simulink subsystem "VL53L_Sensor"  (R2022b)
settings: Solver=VariableStepAuto  StartTime=0.0  StopTime=10.0  RelTol=1e-3
undefined symbols (not defined in the file): K_cc, x
libraries: arduinosensorlib x2
settings Model: Creator=dar.io  LastModifiedBy=dar.io

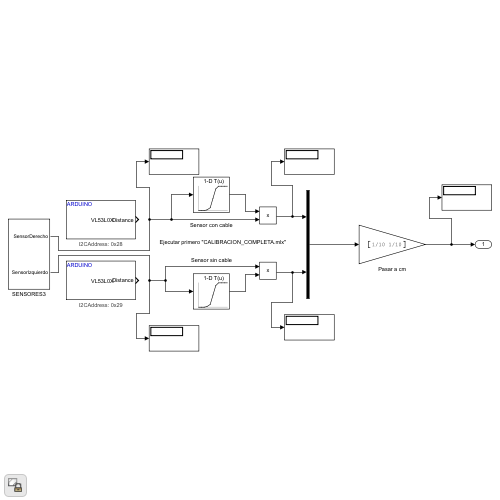
[thumbnail: Simulink's stored preview of the top-level diagram]
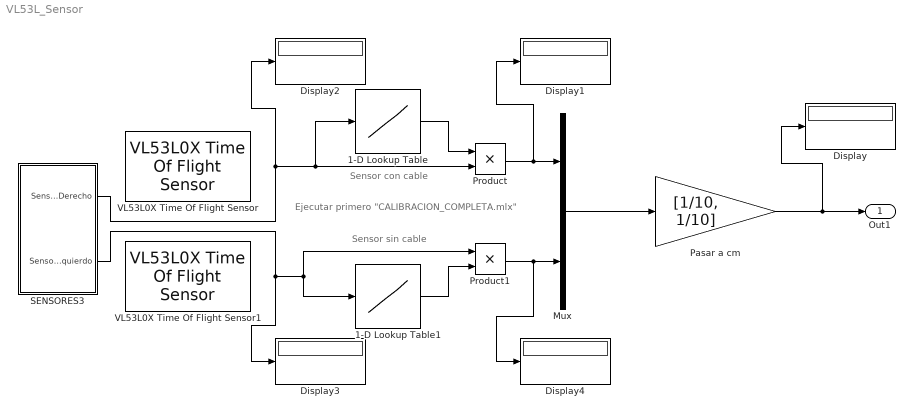
== system VL53L_Sensor ==
  note: Ejecutar primero "CALIBRACION_COMPLETA.mlx"
  note: Sensor sin cable
  note: Sensor con cable
  1-D Lookup Table : Lookup_n-D  NumberOfTableDimensions=1  BreakpointsForDimension1=x  Table=K_cc  ExtrapMethod=Clip  InternalRulePriority=Speed  RndMeth=Simplest
  1-D Lookup Table1 : Lookup_n-D  NumberOfTableDimensions=1  BreakpointsForDimension1=x  Table=K_cc  ExtrapMethod=Clip  InternalRulePriority=Speed  RndMeth=Simplest
  Display{,1..4} (5 alike) : Display
  Mux : Mux  Inputs=2
  Pasar a cm : Gain  Gain=[1/10, 1/10]
  Product : Product
  Product1 : Product
  SENSORES3 : Subsystem
  VL53L0X Time Of Flight Sensor : arduinosensorlib/VL53L0X Time Of Flight Sensor  I2CAddress=0x28  BitRate=1000000  RangingMode=Default  SampleTime=-1
      settings: AttributesFormatString=I2CAddress: %<I2CAddress>
  VL53L0X Time Of Flight Sensor1 : arduinosensorlib/VL53L0X Time Of Flight Sensor  I2CAddress=0x29  BitRate=1000000  RangingMode=Default  SampleTime=-1
      settings: AttributesFormatString=I2CAddress: %<I2CAddress>
  Out1 : Outport
  wires:
  Mux/1 -> Pasar a cm/1
  Pasar a cm/1 -> Out1/1, Display/1
  1-D Lookup Table/1 -> Product/1
  1-D Lookup Table1/1 -> Product1/2
  Product/1 -> Display1/1, Mux/1
  SENSORES3/1(SensorDerecho) -> Display2/1, Product/2, 1-D Lookup Table/1
  SENSORES3/2(SensorIzquierdo) -> 1-D Lookup Table1/1, Product1/1, Display3/1
  Product1/1 -> Display4/1, Mux/2

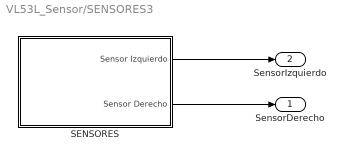
== system VL53L_Sensor/SENSORES3 ==
  SENSORES : Subsystem
  SensorDerecho : Outport  VectorParamsAs1DForOutWhenUnconnected=off
  SensorIzquierdo : Outport  Port=2  VectorParamsAs1DForOutWhenUnconnected=off
  wires:
  SENSORES/1(Sensor Izquierdo) -> SensorIzquierdo/1
  SENSORES/2(Sensor Derecho) -> SensorDerecho/1

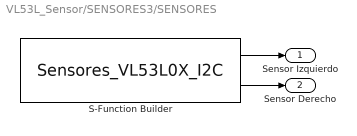
== system VL53L_Sensor/SENSORES3/SENSORES ==
  S-Function Builder : S-Function  InitFcn=try, set_param(gcb,'FunctionName','Sensores_VL53L0X_I2C'), end  FunctionName=Sensores_VL53L0X_I2C  SFunctionModules=Sensores_VL53L0X_I2C_wrapper  SFunctionDeploymentMode=off  EnableBusSupport=off  mask(S-Function Builder){}
      mask help: Simulink:masks:SFunctionBuilder_MD
      mask init:
      | val = [[.9  0.75 0.75 1 1 .9 .9 1]',[1 1 0.75 0.75 .9 .9 1 .9]'];try , sys = get_param(gcb,'SfunBuilderFcnName');if isempty(sys), sys = get_param(gcb,'FunctionName'); end,catch, sys = get_param(gcb,'FunctionName'); end
      settings: CopyFcn=set_param(gcbh,'LinkStatus','none')  PreSaveFcn=try, set_param(gcb,'FunctionName','Sensores_VL53L0X_I2C'), end  OpenFcn=sfunctionwizard(gcbh)
      mask Display: plot(val(:,1),val(:,2)),disp(sys), port_label('output',1,'Sensor1'), port_label('output',2,'Sensor2')
  Sensor Izquierdo : Outport  VectorParamsAs1DForOutWhenUnconnected=off
  Sensor Derecho : Outport  Port=2  VectorParamsAs1DForOutWhenUnconnected=off
  wires:
  S-Function Builder/1 -> Sensor Izquierdo/1
  S-Function Builder/2 -> Sensor Derecho/1
